simulink model "thyristor_1phase_bridge_inductive_load"  (R2015a)
settings: Solver=ode45  StartTime=0.0  StopTime=0.03  MaxStep=1/1000  RelTol=1e-3
libraries: powerlib x9, simulink x2
settings Model: Creator=Windows 10  LastModifiedBy=Windows 10

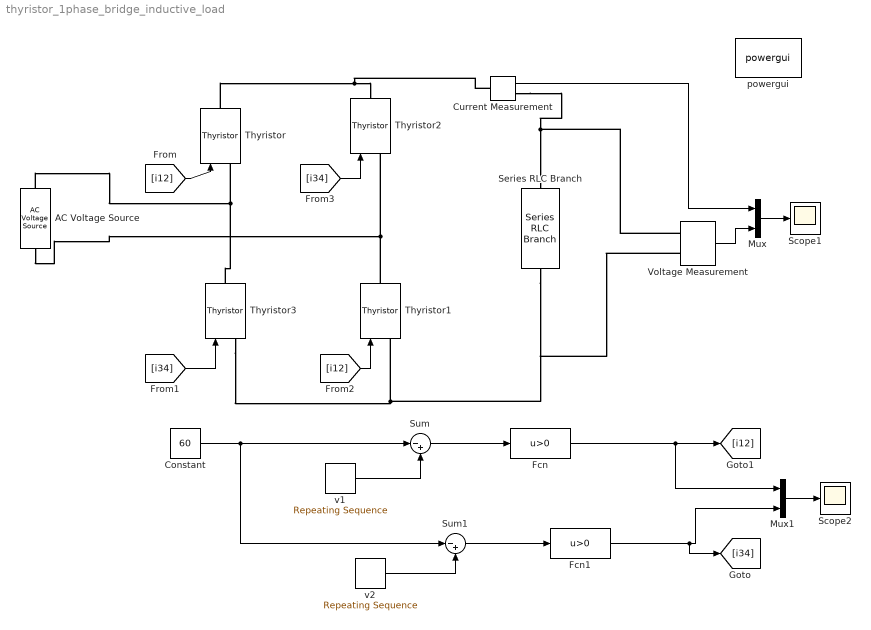
== system thyristor_1phase_bridge_inductive_load ==
  AC Voltage Source : powerlib/Electrical Sources/AC Voltage Source  Amplitude=100*3  Phase=0  Frequency=60-10  SampleTime=0  Measurements=None
  Constant : Constant  Value=60
  Current Measurement : powerlib/Measurements/Current Measurement  PhasorSimulation=off  OutputType=Complex  PSBequivalent=0
  Fcn : Fcn  Expr=u>0
  Fcn1 : Fcn  Expr=u>0
  Mux : Mux  Inputs=2
  Mux1 : Mux  Inputs=2
  Scope1 : Scope
  Scope2 : Scope
  Series RLC Branch : powerlib/Elements/Series RLC Branch  LConnTagsString=__new0  RConnTagsString=__new0  BranchType=RL  Resistance=2  Inductance=4*1e-3  SetiL0=off  InitialCurrent=0  Capacitance=1e-6  Setx0=off  InitialVoltage=0  Measurements=None
  Sum : Sum  Inputs=|-+
  Sum1 : Sum  Inputs=|-+
  Thyristor{,1..3} (4 alike) : powerlib/Power Electronics/Thyristor  Ron=0.001  Lon=0  Vf=0.8  IC=0  Rs=500  Cs=250e-9  Measurements=off
  Voltage Measurement : powerlib/Measurements/Voltage Measurement  PhasorSimulation=off  OutputType=Complex  PSBequivalent=0
  powergui : powerlib/powergui  Priority=1  SimulationMode=Continuous  SolverType=Tustin/Backward Euler (TBE)  SampleTime=50e-6  frequency=60  SPID=off  DisableSnubberDevices=off  DisableRonSwitches=off  DisableVfSwitches=off  SwTol=0  DisplayEquations=off  Interpol=off  methode=off  Ts=100  FunctionMessages=off  echomessages=off  HookPort=off  EnableUseOfTLC=off  x0status=blocks  frequencyindice=50  Pbase=100e6  ErrMax=1e-4  Iterations=50  UnitsV=kV  UnitsW=MW  buscounter=0  RestoreLinks=warning  ResistiveCurrentMeasurement=off  Frange=[0:2:500]  Ylog=off  Xlog=on  ShowGrid=off  save=off  variable=ZData  structure=0  ZoomFFT=off  StartTime=0.0  cycles=1  DisplayStyle=1  fundamental=60  FreqAxis=off  MaxFrequency=1000  frequencyindicesteady=1  RmsSteady=1  display=off
  v1 : simulink/Sources/Repeating Sequence  rep_seq_t=[0 10 10.00001 20]*1e-3  rep_seq_y=[0 180 -180 0]
  v2 : simulink/Sources/Repeating Sequence  rep_seq_t=[0 20 20.00001]*1e-3  rep_seq_y=[-180 180 -180]
  wires:
  v1/1 -> Sum/2
  Voltage Measurement/1 -> Mux/2
  Current Measurement/1 -> Mux/1
  Mux/1 -> Scope1/1
  Constant/1 -> Sum1/1, Sum/1
  v2/1 -> Sum1/2
  Sum/1 -> Fcn/1
  Sum1/1 -> Fcn1/1
  Fcn1/1 -> [i34], Mux1/2
  Fcn/1 -> [i12], Mux1/1
  [i34] -> Thyristor2/1
  [i12] -> Thyristor/1
  [i34] -> Thyristor3/1
  [i12] -> Thyristor1/1
  Mux1/1 -> Scope2/1
  connections:
  Thyristor/RConn1 -- Current Measurement/LConn1 -- Thyristor2/RConn1
  Thyristor3/LConn1 -- Series RLC Branch/RConn1 -- Voltage Measurement/LConn2 -- Thyristor1/LConn1
  Thyristor3/RConn1 -- AC Voltage Source/RConn1 -- Thyristor/LConn1
  Thyristor1/RConn1 -- AC Voltage Source/LConn1 -- Thyristor2/LConn1
  Current Measurement/RConn1 -- Series RLC Branch/LConn1 -- Voltage Measurement/LConn1
